simulink model "GFo_5bus"  (R2017b)
settings: Solver=ode1  StartTime=0.0  StopTime=4  FixedStep=Time_Step  MaxStep=0.04  RelTol=1e-3  EnableMultiTasking=on
PreLoadFcn:
  | Init_5bus;
InitFcn:
  | Init_5bus;
undefined symbols (not defined in the file): D1, Delta, Time_Step, VSC01_Delta_P_Time_Step, VSC01_Delta_P_Value
libraries: powerlib x19, GFo_Lib x2
Description:
  | Copyright 2008-2017 The MathWorks, Inc.
settings Model: Creator=MathWorks  LastModifiedBy=Frederic_Colas
settings DataIOCC: LimitDataPoints=on  SaveFormat=Array  SignalLoggingSaveFormat=ModelDataLogs
settings OptimizationCC: ExpressionDepthLimit=2147483647  LifeSpan=inf
settings DebuggingCC: UnderspecifiedInitializationDetection=Classic  MergeDetectMultiDrivingBlocksExec=none  SolverPrmCheckMsg=warning  FcnCallInpInsideContextMsg=warning  UnconnectedInputMsg=none  UnconnectedOutputMsg=none  UnconnectedLineMsg=none  StateNameClashWarn=warning  SFUnexpectedBacktrackingDiag=warning  SFNoUnconditionalDefaultTransitionDiag=warning  SFExecutionAtInitializationDiag=none
settings HardwareCC: ProdBitPerPointer=32  ProdBitPerSizeT=32  ProdBitPerPtrDiffT=32  ProdLargestAtomicFloat=None  ProdIntDivRoundTo=Undefined  ProdEndianess=Unspecified  ProdWordSize=32  ProdHWDeviceType=32-bit Generic
settings ModelReferenceCC: PropagateSignalLabelsOutOfModel=off
settings CodeAppCC: StateflowObjectComments=on
settings GRTTargetCC: TargetLangStandard=C89/C90 (ANSI)  GeneratePreprocessorConditionals=Disable all  CombineOutputUpdateFcns=off  GRTInterface=on
settings ConfigComp: CovMetricSettings=dw  CovHtmlReporting=on  CovSaveCumulativeToWorkspaceVar=on  CovSaveSingleToWorkspaceVar=on  CovExternalEMLEnable=off  CovSFcnEnable=off
settings SimscapeCC: SimscapeNormalizeSystem=off

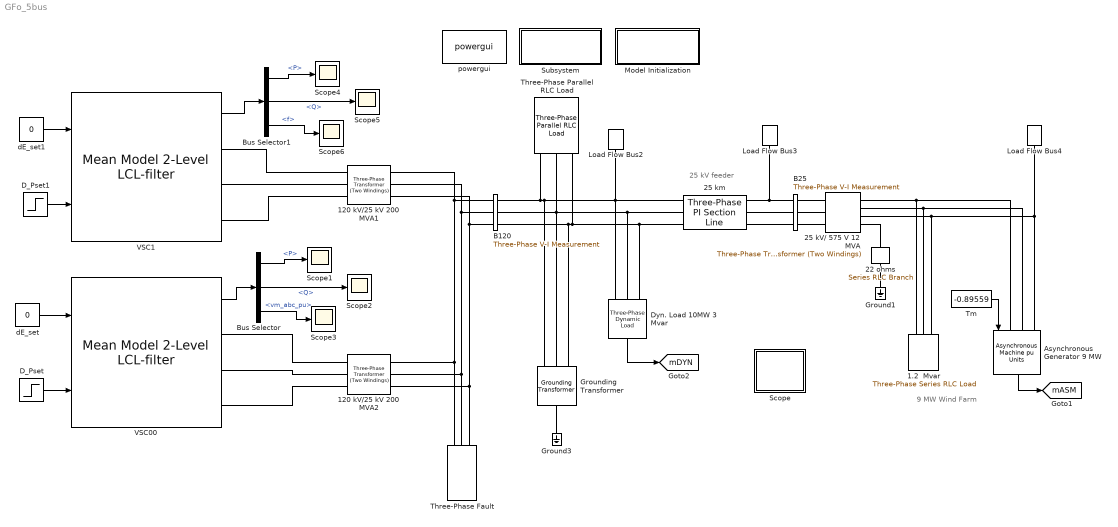
== system GFo_5bus ==
  note: 9 MW Wind Farm
  note: 25 kV feeder
  1.2  Mvar : powerlib/Elements/Three-Phase Series RLC Load  LConnTagsString=A|B|C  Configuration=Delta  NominalVoltage=575  Vabc=[1e3 1e3 1e3]  Vabcp=[1e3 1e3 1e3]  NominalFrequency=60  UnbalancedPower=off  ActivePower=1.2e6/50  InductivePower=0  CapacitivePower=1.2e6  Pabc=[10e3 9e3 11e3]  QLabc=[100 90 110]  QCabc=[100 90 110]  Pabcp=[10e3 9e3 11e3]  QLabcp=[100 90 110]  QCabcp=[100 90 110]  Measurements=None  LoadType=constant Z
  120 kV/25 kV 200 MVA1 : powerlib/Elements/Three-Phase Transformer (Two Windings)  Winding1Connection=Yg  Winding2Connection=Delta (D1)  CoreType=Three single-phase transformers  SetSaturation=off  Hysteresis=off  DataFile='basic_model'  SetInitialFlux=off  Measurements=None  UNITS=pu  NominalPower=[200e6 60 ]  Winding1="[ 120e3  0.002    0.06 ]"  Winding2="[ 25e3  0.002  0.06]"  Rm=500  Lm=500  L0=0.5  Saturation="[ 0,0  ;  0.005,1.2  ;  1.0,1.4 ]"  InitialFluxes=[ 0.8 , -0.8 , 0.7 ]  MoreParameters=off  BreakLoop=off  DataType=off  TransfoNumber=0
  120 kV/25 kV 200 MVA2 : powerlib/Elements/Three-Phase Transformer (Two Windings)  Winding1Connection=Yg  Winding2Connection=Delta (D1)  CoreType=Three single-phase transformers  SetSaturation=off  Hysteresis=off  DataFile='basic_model'  SetInitialFlux=off  Measurements=None  UNITS=pu  NominalPower=[200e6 60 ]  Winding1="[ 120e3  0.002    0.06 ]"  Winding2="[ 25e3  0.002  0.06]"  Rm=500  Lm=500  L0=0.5  Saturation="[ 0,0  ;  0.005,1.2  ;  1.0,1.4 ]"  InitialFluxes=[ 0.8 , -0.8 , 0.7 ]  MoreParameters=off  BreakLoop=off  DataType=off  TransfoNumber=0
  "22 ohms " : powerlib/Elements/Series RLC Branch  LConnTagsString=__new0  RConnTagsString=__new0  BranchType=R  Resistance=22  Inductance=1.0  SetiL0=off  InitialCurrent=0  Capacitance=1.0  Setx0=off  InitialVoltage=0  Measurements=None
  25 kV/ 575 V 12 MVA : powerlib/Elements/Three-Phase Transformer (Two Windings)  Winding1Connection=Yg  Winding2Connection=Yn  CoreType=Three single-phase transformers  SetSaturation=off  Hysteresis=off  DataFile='hysteresis'  SetInitialFlux=off  Measurements=None  UNITS=pu  NominalPower="[12e6  60]"  Winding1=[25e3 , 0.025/30 , 0.025]  Winding2=[ 575, 0.025/30 , 0.025]  Rm=500  Lm=inf  L0=0.5  Saturation=[ 0,0 ; 0.0024,1.2 ; 1.0,1.52 ]  InitialFluxes=[ 0.8 , -0.8 , 0.7 ]  MoreParameters=off  BreakLoop=off  DataType=off  TransfoNumber=0
  25 km : powerlib/Elements/Three-Phase PI Section Line  LConnTagsString=a|b|c  RConnTagsString=A|B|C  Frequency=60  Resistances=[0.1153 0.413]  Inductances=[1.05e-3 3.32e-3]  Capacitances=[11.33e-009 5.01e-009]  Length=25
      settings: SourceProductName=Simscape Power Systems
  Asynchronous Generator 9 MW : powerlib/Machines/Asynchronous Machine pu Units  RotorType=Squirrel-cage  PresetModel=No  MechanicalLoad=Torque Tm  ShowDetailedParameters=on  ReferenceFrame=Rotor  Units=pu  MeasurementBus=off  NominalParameters=[6*1.5e6/0.9 575 60]  Stator=[ 0.004843 0.1248]  Rotor=[ 0.004377 0.1791]  Cage1=[0.01909 0.0397]  Cage2=[0.01909 0.0397]  Lm=6.77  Mechanical="[5.04  0  3]"  PolePairs=3  InitialConditions=[-0.00492233 0 1.02886 1.02886 1.02886 -172.901 -292.901 -52.9007]  SimulateSaturation=off  Saturation=[ 0 0 ; 0 0 ]  LoadFlowParameters=0  TsPowergui=0  TsBlock=-1  IterativeModel=Trapezoidal non iterative  IterativeDiscreteModel=Trapezoidal non iterative  Pmec=-9000000
      settings: SourceProductName=Simscape Power Systems  SourceProductBaseCode=PS
  B120 : powerlib/Measurements/Three-Phase V-I Measurement  VoltageMeasurement=phase-to-ground  SetLabelV=on  LabelV=Vabc_B120  Vpu=on  VpuLL=off  CurrentMeasurement=no  SetLabelI=on  LabelI=Iabc_B120  Ipu=off  Pbase=100e6  Vbase=120e3  OutputType=Complex  PhasorSimulation=off  PSBequivalent=0
  B25 : powerlib/Measurements/Three-Phase V-I Measurement  VoltageMeasurement=phase-to-ground  SetLabelV=on  LabelV=Vabc_B25  Vpu=on  VpuLL=off  CurrentMeasurement=yes  SetLabelI=on  LabelI=Iabc_B25  Ipu=on  Pbase=10e6  Vbase=25e3  OutputType=Complex  PhasorSimulation=off  PSBequivalent=0
  Bus Selector : BusSelector  OutputSignals=control.P,control.Q,control.vm.vm_abc_pu
  Bus Selector1 : BusSelector  OutputSignals=control.P,control.Q,control.f
  D_Pset : Step  Time=VSC01_Delta_P_Time_Step  After=VSC01_Delta_P_Value  SampleTime=0
  D_Pset1 : Step  Time=VSC01_Delta_P_Time_Step  After=VSC01_Delta_P_Value*0  SampleTime=0
  Dyn. Load 10MW 3 Mvar : powerlib/Elements/Three-Phase Dynamic Load  NominalVoltage=[ 25e3 60 ]  ActiveReactivePowers=[1e+07 3e+06]  PositiveSequence=[0.994477 -30.2373]  ExternalControl=off  NpNq=[1.5 2.5]  TimeConstants="[0  0  0  0]"  MinimumVoltage=0.7  Tfilter=1e-4  LoadFlowParameters=[4,0,0,0,0]
      settings: SourceProductName=Simscape Power Systems  SourceProductBaseCode=PS
  Ground1 : powerlib/Elements/Ground  LConnTagsString=a
  Ground3 : powerlib/Elements/Ground  LConnTagsString=a
  "Grounding Transformer " : powerlib/Elements/Grounding Transformer   UNITS=SI  NominalPower="[100e6   60]"  NominalVoltage=25e3  ZeroSequenceImpedance_pu=[0.025 0.75]  MagnetizationBranch_pu=[500 500]  ZeroSequenceImpedance_SI=[0.15625 4.6875]  MagnetizationBranch_SI=[3125 3125]  Measurements=None
      settings: SourceProductName=Simscape Power Systems  SourceProductBaseCode=PS
  Load Flow Bus2 : powerlib/Measurements/Load Flow Bus  LConnTagsString=a  Phases=single  Connectors=on one side  ID=B25_1  Vbase=25e3  Vref=1  Vangle=0  VLF=0.9945  VLFb=1  VLFc=1  angleLF=-30.24  angleLFb=0  angleLFc=0
      settings: AttributesFormatString=%<ID>\n%<Vbase>V\n%<VLF>pu\n%<angleLF>deg.  SourceProductName=Simscape Power Systems
  Load Flow Bus3 : powerlib/Measurements/Load Flow Bus  LConnTagsString=a  Phases=single  Connectors=on one side  ID=B25_2  Vbase=25e3  Vref=1  Vangle=0  VLF=0.9662  VLFb=1  VLFc=1  angleLF=-20.9  angleLFb=0  angleLFc=0
      settings: AttributesFormatString=%<ID>\n%<Vbase>V\n%<VLF>pu\n%<angleLF>deg.  SourceProductName=Simscape Power Systems
  Load Flow Bus4 : powerlib/Measurements/Load Flow Bus  LConnTagsString=a  Phases=single  Connectors=on one side  ID=B575  Vbase=575  Vref=1  Vangle=0  VLF=0.953  VLFb=1  VLFc=1  angleLF=-18.58  angleLFb=0  angleLFc=0
      settings: AttributesFormatString=%<ID>\n%<Vbase>V\n%<VLF>pu\n%<angleLF>deg.  SourceProductName=Simscape Power Systems
  Model Initialization : Subsystem  mask(Model Functions){InitFcnX=Init_5bus;, prel=on, posl=off, inif=on, strf=off}
      mask prompts: InitFcnX "Initialisation"; prel "Preload Function"; posl "PostLoad Function"; inif "InitFcn"; strf "StartFcn"
      mask init:
      | currentBlock = gcb;
      | root = bdroot(currentBlock);
      | 
      | if ~strcmp(get_param(root,'BlockDiagramType'),'library')
      |     if prel==1
      |         set_param(root, 'PreLoadFcn', InitFcnX);
      |     else
      |         set_param(root, 'PreLoadFcn', '');
      |     end
      |     if inif==1
      |         set_param(root, 'InitFcn', InitFcnX);
      |     else
      |         set_param(root, 'InitFcn', '');
      |     end
      |     if strf==1
      |         set_param(root, 'StartFcn', InitFcnX);
      |     else
      |         set_param(root, 'StartFcn', '');
      |     end
      |     if posl==1
      |         set_param(root, 'PostLoadFcn', InitFcnX);
      |     else
      |         set_param(root, 'PostLoadFcn', '');
      |     end
      | end
      | 
      | pos = get_param(currentBlock, 'Position');
      | width = pos(3) - pos(1); height = pos(4) - pos(2);
      | txt = [ upper(root) '\n' '- InitFcn. . . . . '  get_param(root, 'InitFcn') ];
      settings: CopyFcn=set_param(gcb,'LinkStatus','none')
      mask Display:
      | %text(5, height*0.5, txt, 'horizontalAlignment', 'left', 'verticalAlignment', 'middle') ;
      | color('blue'),disp('Initialization Function\nParameters')
  Scope : Subsystem
  Scope{1..6} (6 alike) : Scope
  Subsystem : Subsystem
      settings: OpenFcn=LoadFlow_VSC
      mask Display: color('blue'),disp('Update Loadflow')
  Three-Phase Parallel RLC Load : powerlib/Elements/Three-Phase Parallel RLC Load  LConnTagsString=A|B|C  Configuration=Y (grounded)  NominalVoltage=25e3  Vabc=[1e3 1e3 1e3]  Vabcp=[1e3 1e3 1e3]  NominalFrequency=60  UnbalancedPower=off  ActivePower=20e6  InductivePower=0  CapacitivePower=0  Pabc=[10e3 9e3 11e3]  QLabc=[100 90 110]  QCabc=[100 90 110]  Pabcp=[10e3 9e3 11e3]  QLabcp=[100 90 110]  QCabcp=[100 90 110]  Measurements=None  LoadType=constant Z
  Three-Phase Fault : powerlib/Elements/Three-Phase Fault  InitialStates=0  FaultA=on  FaultB=off  FaultC=off  GroundFault=on  SwitchTimes=[ 3 3.1]  External=off  SwitchStatus=NaN  FaultResistance=0.001  GroundResistance=0.001  SnubberResistance=1e6  SnubberCapacitance=inf  Measurements=None
  Tm : Constant  Value=-0.89559
  VSC00 : GFo_Lib/Mean Model 2-Level LCL-filter  fn=fb  Sn=VSC01_Sn  Pn=VSC01_Pn  Udcn=240e3  Un1=VSC01_Un1  Un2=VSC01_Un2  Rt_pu=VSC01_Rt_pu  Lt_pu=VSC01_Lt_pu  Rm_pu=500  Lm_pu=500  Lf_pu=VSC01_Lf_pu  Rf_pu=VSC01_Rf_pu  Cf_pu=VSC01_Cf_pu  Tr_PLL=VSC01_Tr_PLL  Val_Freq_Support=on  Val_gamma=on  R_percent=VSC01_R  Rv=VSC01_Rv  W_TVR=VSC01_W_LF  I_thresh_pu=1  DX_DR=5  Kp_Rvi_pu=0.676  gainpopup=3  wc1=VSC01_wc1  mp1=VSC01_mp1  wc2=VSC01_wc2  mp2=VSC01_mp2  wc3=VSC01_wc3  mp3=VSC01_mp3  T1=VSC01_T1  T2=VSC01_T2  LFpopup=PQ  P0=0.099988  Q0=4.4019e-07  V0=0.99461  Theta0=0.27737  innercontrol=1  Kp_i=0.73  Ki_i=1.19  Kp_v=0.52  Ki_v=1.16  Kffv=1  Kffi=1  I_max=1.25
      settings: SourceProductName=VSC4SPS
  VSC1 : GFo_Lib/Mean Model 2-Level LCL-filter  fn=fb  Sn=VSC01_Sn  Pn=VSC01_Pn  Udcn=240e3  Un1=VSC01_Un1  Un2=VSC01_Un2  Rt_pu=VSC01_Rt_pu  Lt_pu=VSC01_Lt_pu  Rm_pu=500  Lm_pu=500  Lf_pu=VSC01_Lf_pu  Rf_pu=VSC01_Rf_pu  Cf_pu=VSC01_Cf_pu  Tr_PLL=VSC01_Tr_PLL  Val_Freq_Support=on  Val_gamma=on  R_percent=VSC01_R  Rv=VSC01_Rv  W_TVR=VSC01_W_LF  I_thresh_pu=1  DX_DR=5  Kp_Rvi_pu=0.676  gainpopup=3  wc1=VSC01_wc1  mp1=VSC01_mp1  wc2=VSC01_wc2  mp2=VSC01_mp2  wc3=VSC01_wc3  mp3=VSC01_mp3  T1=VSC01_T1  T2=VSC01_T2  LFpopup=Swing  P0=0.049086  Q0=0.061202  V0=1  Theta0=0  innercontrol=1  Kp_i=0.73  Ki_i=1.19  Kp_v=0.52  Ki_v=1.16  Kffv=1  Kffi=1  I_max=1.25
      settings: SourceProductName=VSC4SPS
  dE_set : Constant  Value=0
  dE_set1 : Constant  Value=0
  powergui : powerlib/powergui  Priority=1  SimulationMode=Discrete  SampleTime=Time_Step  frequency=60  Iterations=50  frequencyindice=60  Pbase=1000e6  ErrMax=0.0001  UnitsV=kV  UnitsW=MW  buscounter=0  FunctionMessages=off  echomessages=off  EnableUseOfTLC=off  CurrentSourceSwitches=off  DisableSnubberDevices=off  DisableRonSwitches=off  DisableVfSwitches=off  DisplayEquations=off  SolverType=Tustin/Backward Euler (TBE)  Interpol=off  ExternalGateDelay=off  methode=off  Ts=100  x0status=blocks  SPID=on  SwTol=0  HookPort=off  RestoreLinks=warning  ResistiveCurrentMeasurement=off  Frange=[0:2:500]  Ylog=off  Xlog=on  ShowGrid=off  save=off  variable=ZData  structure=0  ZoomFFT=off  StartTime=0.0  cycles=1  DisplayStyle=1  fundamental=60  FreqAxis=off  MaxFrequency=1000  frequencyindicesteady=1  RmsSteady=1  display=off
  tag scope: mASM=global, mDYN=global
  wires:
  Tm/1 -> Asynchronous Generator 9 MW/1
  Asynchronous Generator 9 MW/1 -> [mASM]
  Dyn. Load 10MW 3 Mvar/1 -> [mDYN]
  dE_set/1 -> VSC00/1
  D_Pset/1 -> VSC00/2
  VSC00/1 -> Bus Selector/1
  Bus Selector/1 -> Scope1/1  "<P>"
  Bus Selector/2 -> Scope2/1  "<Q>"
  Bus Selector/3 -> Scope3/1  "<vm_abc_pu>"
  D_Pset1/1 -> VSC1/2
  dE_set1/1 -> VSC1/1
  Bus Selector1/3 -> Scope6/1  "<f>"
  Bus Selector1/2 -> Scope5/1  "<Q>"
  Bus Selector1/1 -> Scope4/1  "<P>"
  VSC1/1 -> Bus Selector1/1
  connections:
  B120/LConn3 -- 120 kV/25 kV 200 MVA1/RConn3 -- 120 kV/25 kV 200 MVA2/RConn3 -- Three-Phase Fault/LConn3
  "Grounding Transformer "/LConn2 -- 25 km/LConn2 -- Dyn. Load 10MW 3 Mvar/LConn2 -- B120/RConn2 -- Three-Phase Parallel RLC Load/LConn2
  Dyn. Load 10MW 3 Mvar/LConn3 -- B120/RConn3 -- "Grounding Transformer "/LConn3 -- Three-Phase Parallel RLC Load/LConn3 -- 25 km/LConn3
  25 km/LConn1 -- B120/RConn1 -- Three-Phase Parallel RLC Load/LConn1 -- "Grounding Transformer "/LConn1 -- Dyn. Load 10MW 3 Mvar/LConn1 -- Load Flow Bus2/LConn1
  25 kV/ 575 V 12 MVA/RConn1 -- Asynchronous Generator 9 MW/LConn1 -- 1.2  Mvar/LConn1
  Asynchronous Generator 9 MW/LConn2 -- 1.2  Mvar/LConn2 -- 25 kV/ 575 V 12 MVA/RConn2
  25 kV/ 575 V 12 MVA/RConn3 -- 1.2  Mvar/LConn3 -- Asynchronous Generator 9 MW/LConn3 -- Load Flow Bus4/LConn1
  25 kV/ 575 V 12 MVA/RConn4 -- "22 ohms "/LConn1
  B25/RConn2 -- 25 kV/ 575 V 12 MVA/LConn2
  B25/LConn3 -- 25 km/RConn3
  B25/RConn3 -- 25 kV/ 575 V 12 MVA/LConn3
  Load Flow Bus3/LConn1 -- B25/LConn1 -- 25 km/RConn1
  Ground1/LConn1 -- "22 ohms "/RConn1
  B25/RConn1 -- 25 kV/ 575 V 12 MVA/LConn1
  B25/LConn2 -- 25 km/RConn2
  120 kV/25 kV 200 MVA1/RConn1 -- B120/LConn1 -- 120 kV/25 kV 200 MVA2/RConn1 -- Three-Phase Fault/LConn1
  B120/LConn2 -- 120 kV/25 kV 200 MVA1/RConn2 -- 120 kV/25 kV 200 MVA2/RConn2 -- Three-Phase Fault/LConn2
  Ground3/LConn1 -- "Grounding Transformer "/RConn1
  VSC1/RConn3 -- 120 kV/25 kV 200 MVA1/LConn3
  VSC1/RConn2 -- 120 kV/25 kV 200 MVA1/LConn2
  VSC1/RConn1 -- 120 kV/25 kV 200 MVA1/LConn1
  VSC00/RConn1 -- 120 kV/25 kV 200 MVA2/LConn1
  VSC00/RConn2 -- 120 kV/25 kV 200 MVA2/LConn2
  VSC00/RConn3 -- 120 kV/25 kV 200 MVA2/LConn3

== system GFo_5bus/Model Initialization ==

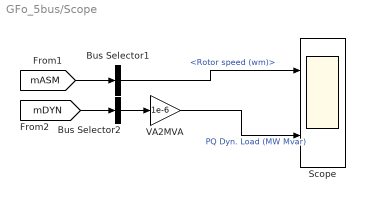
== system GFo_5bus/Scope ==
  Bus Selector1 : BusSelector  OutputSignals=Mechanical.Rotor speed (wm)
  Bus Selector2 : BusSelector  OutputSignals=Active power P (W),Reactive power Q (var)  OutputAsBus=on
  Scope : Scope  NumInputPorts=2
  VA2MVA : Gain  Gain=1e-6
  wires:
  [mASM] -> Bus Selector1/1
  Bus Selector1/1 -> Scope/1  "<Rotor speed (wm)>"
  [mDYN] -> Bus Selector2/1
  Bus Selector2/1 -> VA2MVA/1
  VA2MVA/1 -> Scope/2  "PQ Dyn. Load (MW Mvar)"

== system GFo_5bus/Subsystem ==
